simulink model "Pendulo2019"  (R2019b)
settings: Solver=FixedStepAuto  StartTime=0.0  StopTime=6  FixedStep=0.001  RelTol=1e-3
values from neighbouring files (symbols this model uses):
  g = 9.81    [confusion.m]    (also in main.m; tarea3.m)
  J = m*(l^2)    (= 0.39375)    [confusion.m]    (also in main.m; tarea3.m)
  l = 0.75    [confusion.m]    (also in main.m; tarea3.m)
  m = 0.7    [confusion.m]    (also in main.m; tarea3.m)
undefined symbols (not defined in the file or in its folder): C
settings Model: DataTypeOverride=Double  MinMaxOverflowLogging=ForceOff  Creator=Gamer  LastModifiedBy=mluser

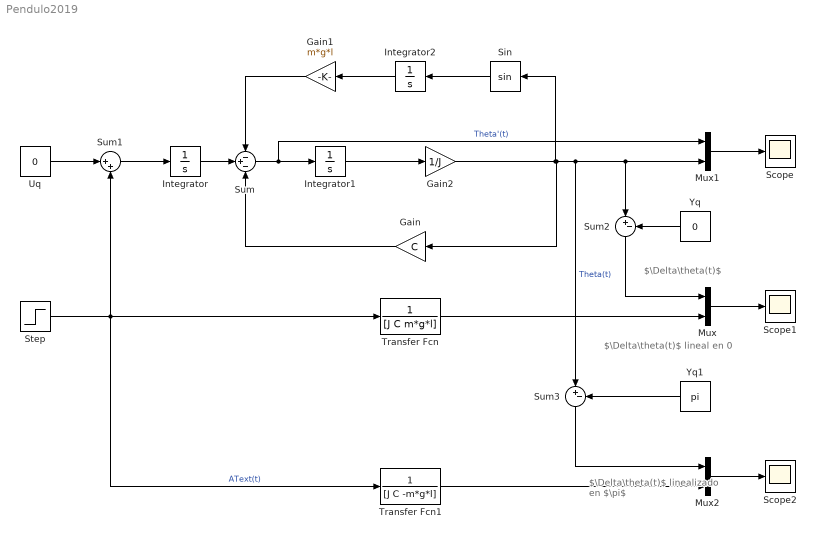
== system Pendulo2019 ==
  note: $\Delta\theta(t)$ lineal en 0
  note: $\Delta\theta(t)$
  note: $\Delta\theta(t)$ linealizado en $\pi$
  Gain : Gain  Gain=C
  Gain1 : Gain  Gain=m*g*l
  Gain2 : Gain  Gain=1/J
  Integrator : Integrator
  Integrator1 : Integrator
  Integrator2 : Integrator
  Mux : Mux  Inputs=2
  Mux1 : Mux  Inputs=2
  Mux2 : Mux  Inputs=2
  Scope : Scope
  Scope1 : Scope
  Scope2 : Scope
  Sin : Trigonometry
  Step : Step  SampleTime=0
  Sum : Sum  Inputs=-+-
  Sum1 : Sum  Inputs=|++
  Sum2 : Sum  Inputs=|+-
  Sum3 : Sum  Inputs=|+-
  Transfer Fcn : TransferFcn  Denominator=[J C m*g*l]
  Transfer Fcn1 : TransferFcn  Denominator=[J C -m*g*l]
  Uq : Constant  Value=0
  Yq : Constant  Value=0
  Yq1 : Constant  Value=pi
  wires:
  Integrator1/1 -> Gain2/1
  Integrator/1 -> Sum/2
  Gain1/1 -> Sum/1
  Gain/1 -> Sum/3
  Sum/1 -> Mux1/1, Integrator1/1  "Theta'(t)"
  Integrator2/1 -> Gain1/1
  Gain2/1 -> Sin/1, Sum3/1, Mux1/2, Sum2/1, Gain/1  "Theta(t)"
  Sin/1 -> Integrator2/1
  Mux/1 -> Scope1/1
  Uq/1 -> Sum1/1
  Sum1/1 -> Integrator/1
  Sum2/1 -> Mux/1
  Yq/1 -> Sum2/2
  Transfer Fcn/1 -> Mux/2
  Step/1 -> Transfer Fcn1/1, Sum1/2, Transfer Fcn/1  "AText(t)"
  Mux1/1 -> Scope/1
  Transfer Fcn1/1 -> Mux2/2
  Mux2/1 -> Scope2/1
  Yq1/1 -> Sum3/2
  Sum3/1 -> Mux2/1
